simulink model "Ext_Springs_CS7"  (Simulink 7.0)
settings: Solver=ode45  SolverMode=SingleTasking  StartTime=0  StopTime=10  FixedStep=0.001  RelTol=1e-3  AbsTol=1e-6
PreLoadFcn:
  | cd Extensions/Simulink/springs
  | spring_e_class
  | cd ../../..
values from neighbouring files (symbols this model uses):
  FS_COMP_TABLE_F = [ ... (first row only)    [spring_e_class.m]
  FS_COMP_TABLE_R = [ ... (first row only)    [spring_e_class.m]
libraries: Solver_SF x1
settings Model: Creator=dhall  LastModifiedBy=ywata  ExtModeTrigMode=oneshot  ExtModeArmWhenConnect=off
settings DataIOCC: LimitDataPoints=off  SignalLoggingName=sigsOut
settings OptimizationCC: BooleanDataType=off  InlineInvariantSignals=on  InitFltsAndDblsToZero=off
settings DebuggingCC: SaveWithParameterizedLinksMsg=none  SignalResolutionControl=TryResolveAllWithWarning  SolverPrmCheckMsg=none  MultiTaskDSMMsg=warning  MultiTaskCondExecSysMsg=none  StrictBusMsg=None
settings HardwareCC: TargetUnknown=on
settings RTWCC: TemplateMakefile=grt_vc.tmf  IncludeERTFirstTime=on
settings GRTTargetCC: TargetFcnLib=ansi_tfl_tmw.mat

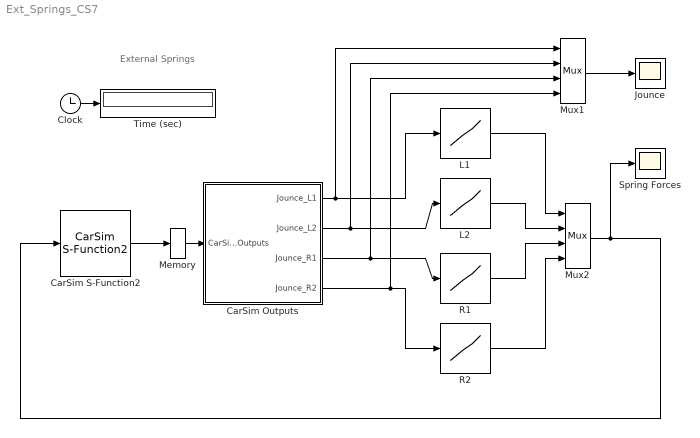
== system Ext_Springs_CS7 ==
  note: External Springs
  CarSim Outputs : Subsystem
  CarSim S-Function2 : Solver_SF/CarSim S-Function2  Priority=1  VehicleCode=???
      settings: AttributesFormatString=Vehicle Code: %<VehicleCode>
  Clock : Clock
      settings: Decimation=10
  Jounce : Scope
      settings: TickLabels=on  TimeRange=7  YMin=-60  YMax=40  DataFormat=Array  SampleTime=100
  L1 : Lookup  InputValues=FS_COMP_TABLE_F(:,1)  Table=FS_COMP_TABLE_F(:,2)  OutDataType=sfix(16)  OutScaling=2^0  SaturateOnIntegerOverflow=on
  L2 : Lookup  InputValues=FS_COMP_TABLE_R(:,1)  Table=FS_COMP_TABLE_R(:,2)  OutDataType=sfix(16)  OutScaling=2^0  SaturateOnIntegerOverflow=on
  Memory : Memory
  Mux1 : Mux
  Mux2 : Mux
  R1 : Lookup  InputValues=FS_COMP_TABLE_F(:,1)  Table=FS_COMP_TABLE_F(:,2)  OutDataType=sfix(16)  OutScaling=2^0  SaturateOnIntegerOverflow=on
  R2 : Lookup  InputValues=FS_COMP_TABLE_R(:,1)  Table=FS_COMP_TABLE_R(:,2)  OutDataType=sfix(16)  OutScaling=2^0  SaturateOnIntegerOverflow=on
  Spring Forces : Scope
      settings: TickLabels=on  TimeRange=7  YMin=2000  YMax=7000  DataFormat=Array  SampleTime=100
  Time (sec) : Display
      settings: Format=bank  Decimation=100
  wires:
  Mux1/1 -> Jounce/1
  CarSim Outputs/1(Jounce_L1) -> L1/1, Mux1/1
  CarSim Outputs/2(Jounce_L2) -> L2/1, Mux1/2
  CarSim Outputs/3(Jounce_R1) -> R1/1, Mux1/3
  CarSim Outputs/4(Jounce_R2) -> R2/1, Mux1/4
  L1/1 -> Mux2/1
  L2/1 -> Mux2/2
  R1/1 -> Mux2/3
  R2/1 -> Mux2/4
  CarSim S-Function2/1 -> Memory/1
  Clock/1 -> Time (sec)/1
  Mux2/1 -> Spring Forces/1, CarSim S-Function2/1
  Memory/1 -> CarSim Outputs/1(CarSim Outputs)

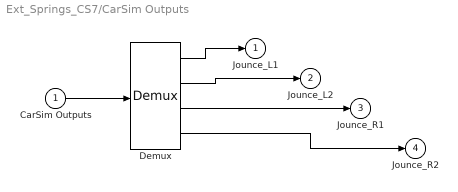
== system Ext_Springs_CS7/CarSim Outputs ==
  CarSim Outputs : Inport  OutDataType=sfix(16)  OutScaling=2^0
  Demux : Demux
  Jounce_L1 : Outport  InitialOutput=0
  Jounce_L2 : Outport  Port=2  InitialOutput=0
  Jounce_R1 : Outport  Port=3  InitialOutput=0
  Jounce_R2 : Outport  Port=4  InitialOutput=0
  wires:
  CarSim Outputs/1 -> Demux/1
  Demux/1 -> Jounce_L1/1
  Demux/2 -> Jounce_L2/1
  Demux/3 -> Jounce_R1/1
  Demux/4 -> Jounce_R2/1
